simulink model "PID_controller_implementation_RHZ"  (R2023b)
settings: Solver=VariableStepAuto  StartTime=0.0  StopTime=10.0  RelTol=1e-3
settings Model: Creator=suvo  LastModifiedBy=suvo

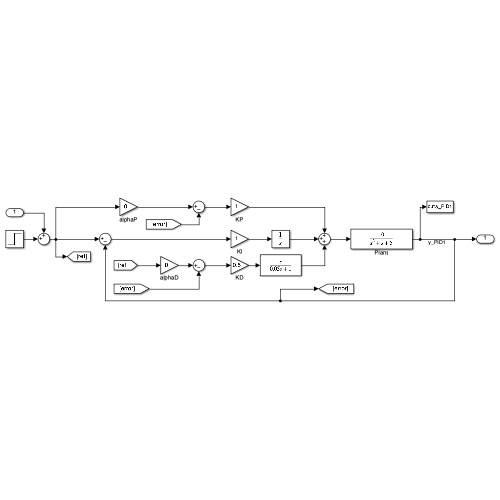
[thumbnail: Simulink's stored preview of the top-level diagram]
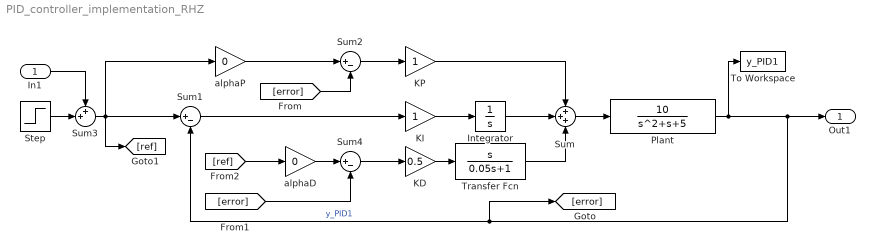
== system PID_controller_implementation_RHZ ==
  In1 : Inport
  Integrator : Integrator
  KD : Gain  Gain=0.5
  KI : Gain
  KP : Gain
  Plant : TransferFcn  Numerator=10  Denominator=[1 1 5]
  Step : Step  SampleTime=0
  Sum : Sum  Inputs=+++
  Sum1 : Sum  Inputs=|+-
  Sum2 : Sum  Inputs=|+-
  Sum3 : Sum  Inputs=++|
  Sum4 : Sum  Inputs=|+-
  To Workspace : ToWorkspace  VariableName=y_PID1  SaveFormat=Timeseries  SampleTime=-1
  Transfer Fcn : TransferFcn  Numerator=[1 0]  Denominator=[0.05 1]
  alphaD : Gain  Gain=0
  alphaP : Gain  Gain=0
  Out1 : Outport
  wires:
  Sum2/1 -> KP/1
  KD/1 -> Transfer Fcn/1
  [ref] -> alphaD/1
  Integrator/1 -> Sum/2
  Sum1/1 -> KI/1
  KP/1 -> Sum/1
  Sum4/1 -> KD/1
  In1/1 -> Sum3/1
  [error] -> Sum4/2
  Sum/1 -> Plant/1
  alphaD/1 -> Sum4/1
  Step/1 -> Sum3/2
  [error] -> Sum2/2
  KI/1 -> Integrator/1
  Plant/1 -> To Workspace/1, Out1/1, Sum1/2, [error]  "y_PID1"
  Transfer Fcn/1 -> Sum/3
  Sum3/1 -> alphaP/1, Sum1/1, [ref]
  alphaP/1 -> Sum2/1
